simulink model "PippoSchema"  (R2022b)
settings: Solver=VariableStepAuto  StartTime=0.0  StopTime=2  RelTol=1e-3
settings Model: Creator=Stefano  LastModifiedBy=stefanopanzieri
settings SolverCC: AlgebraicLoopSolver=TrustRegion
settings OptimizationCC: ReuseModelBlockBuffer=on
settings DebuggingCC: UnconnectedInputMsg=warning  UnconnectedOutputMsg=warning  UnconnectedLineMsg=warning
settings ModelReferenceCC: EnableRefExpFcnMdlSchedulingChecks=on
settings SFSimCC: CustomCodeUndefinedFunction=UseInterfaceOnly
settings RTWCC: DLArmComputeVersion=19.05

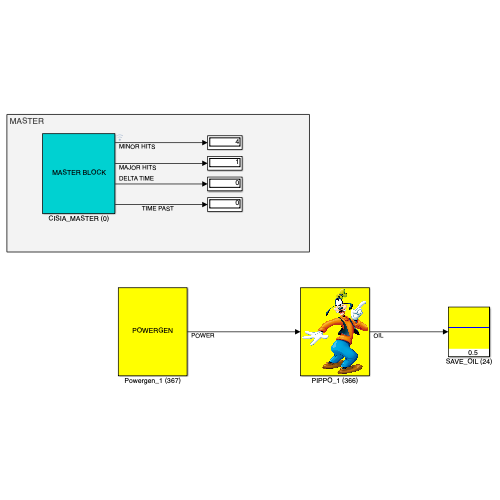
[thumbnail: Simulink's stored preview of the top-level diagram]
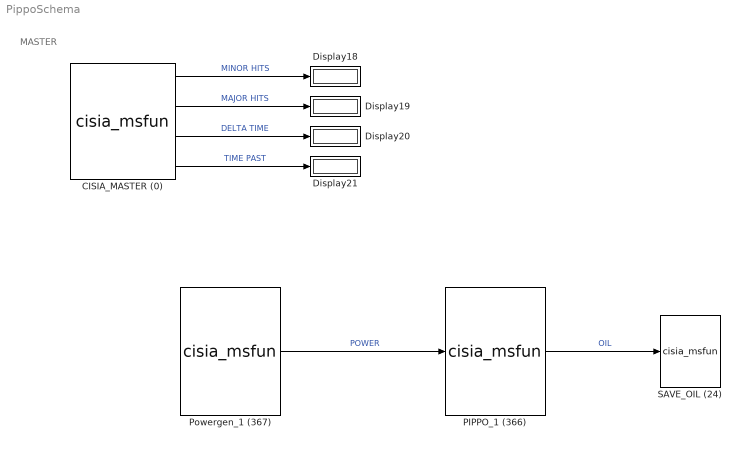
== system PippoSchema ==
  note: MASTER
  CISIA_MASTER (0) : M-S-Function  FunctionName=cisia_msfun  Parameters=Parameter1, Parameter2, Parameter3, resources, Parameter4, Parameter5, Parameter6, Parameter7, Parameter8, Parameter9,Parameter11  mask(S-function:msfcn_unit_delay){Parameter1='CISIA_MASTER', Parameter2=1, Parameter3='SistemiIoT', resources=off, Parameter4=on, Parameter5=off, Parameter6=off, Parameter7=off, Parameter8=0.001, Parameter9=off, Parameter11=on}
      mask prompts: Parameter1 "entity name"; Parameter2 "sampling time"; Parameter3 "project"; resources "Save status at each major hit"; Parameter4 "Show Operative Levels with colors"; Parameter5 "Load Entities from file"; Parameter6 "Load Start from Mask"; Parameter7 "Real Time"; Parameter8 "Real Time Hit (sec)"; Parameter9 "Skip saving"; Parameter11 "Show unconnected"
      mask help: This is a level-2 MATLAB file S-function which demonstrates CISIA entity
      mask Display: disp('MASTER BLOCK')
  Display{18..21} (4 alike) : Display
  PIPPO_1 (366) : M-S-Function  FunctionName=cisia_msfun  Parameters=Parameter1, Parameter2, Parameter3, resources, Parameter10, codeupdate, step_received, step_computed, dynamic_computed, step_sended, id_entity, id_project, id_type, name_type, color  mask(S-function:msfcn_unit_delay){Parameter1='PIPPO_1', Parameter2=1, Parameter3='', resources=|, Parameter10=off, codeupdate=off, step_received=Operative_Level=min([POWER  1-Mechanical_Fault]);, step_computed=, dynamic_computed=, step_sended=OIL=Operative_Level;, id_entity=366, id_project=6, id_type=100, name_type=PIPPO, color=#FFFFFF}
      mask resources=|
      | *** INPUT RESOURCES ***
      | NUM_INPUTS 1
      | POWER (1)
      |
      | *** STATE VARIABLES ***
      | NUM_VARIABLES 2
      | Operative_Level(NUMERIC)(1)(1)
      | Mechanical_Fault(NUMERIC)(1)(0)
      |
      | *** OUTPUT RESOURCES ***
      | NUM_OUTPUTS 1
      | OIL (1)
      mask prompts: Parameter1 "entity name"; Parameter2 "sampling time"; Parameter3 "project"; resources "input resources and state variables"; Parameter10 "Bring state variables to output"; codeupdate "update code from mask"
      mask help: This is a level-2 MATLAB file S-function which demonstrates CISIA entity
      mask DialogControl Container1 Prompt: All parameters
      mask Display: image('Icons/PIPPO.png')
  Powergen_1 (367) : M-S-Function  FunctionName=cisia_msfun  Parameters=Parameter1, Parameter2, Parameter3, resources, Parameter10, codeupdate, step_received, step_computed, dynamic_computed, step_sended, id_entity, id_project, id_type, name_type, color  mask(S-function:msfcn_unit_delay){Parameter1='Powergen_1', Parameter2=1, Parameter3='', resources=|, Parameter10=off, codeupdate=off, step_received=Operative_Level=1-Physical_Fault;, step_computed=, dynamic_computed=, step_sended=POWER=Operative_Level;, id_entity=367, id_project=6, id_type=101, name_type=POWERGEN, color=#FFFFFF}
      mask resources=|
      | *** INPUT RESOURCES ***
      | NUM_INPUTS 0
      |
      | *** STATE VARIABLES ***
      | NUM_VARIABLES 2
      | Operative_Level(NUMERIC)(1)(1)
      | Physical_Fault(NUMERIC)(1)(0.5)
      |
      | *** OUTPUT RESOURCES ***
      | NUM_OUTPUTS 1
      | POWER (1)
      mask prompts: Parameter1 "entity name"; Parameter2 "sampling time"; Parameter3 "project"; resources "input resources and state variables"; Parameter10 "Bring state variables to output"; codeupdate "update code from mask"
      mask help: This is a level-2 MATLAB file S-function which demonstrates CISIA entity
      mask DialogControl Container1 Prompt: All parameters
      mask Display: disp('POWERGEN')
  SAVE_OIL (24) : M-S-Function  FunctionName=cisia_msfun  Parameters=Parameter1, Parameter2, Parameter3, Parameter4,Parameter5,Parameter6,Parameter7  mask(S-function:msfcn_unit_delay){Parameter1='SAVE_OIL', Parameter2=1, Parameter3='SistemiIoT', Parameter4=on, Parameter5=[0.5], Parameter6=[1], Parameter7=off}
      mask prompts: Parameter1 "entity name"; Parameter2 "sampling time"; Parameter3 "project"; Parameter4 "display bars"; Parameter5 "values"; Parameter6 "logic"; Parameter7 "display B/W"
      mask help: This is a level-2 MATLAB file S-function which demonstrates CISIA entity
      mask DialogControl Container3 Prompt: Display
      mask Display:
      | display=get_param(gcb, 'Parameter4');
      | greymap=get_param(gcb, 'Parameter7');
      | 
      | if strcmp(display,'on')
      | 
      |     val=str2num(get_param(gcb, 'Parameter5'));
      |     logic=str2num(get_param(gcb, 'Parameter6'));
      |     n=length(val);
      | 
      |     val2=val;
      |     l=length(logic);
      |     if l>0
      |         for i=1:l
      |             if logic(i)==-1
      |                 val2(i)=1-val2(i);
      |             end
      |         end
      |     end
      | 
      | 
      | 
      | 
      |     if strcmp(greymap,'on')
      |         val_r=round(val2*50)+1;
      |         colormap=gray(60);
      |         color2=[0 0 0];
      |     else
      |         val_r=round(val2*20)+1;
      |         colormap=hsv(60);
      |         color2=[0 0 1];
      |     end
      | 
      |     patch([0 0 n n], [0 -0.2 -0.2 0], [1 1 1]);
      | 
      |     for i=1:n
      |         color=colormap(val_r(i),:);
      |         patch([i-1 i-1 i i],[0 1 1 0],color)
      |         patch([i-1 i],[val(i) val(i)],color2)
      | 
      |     end
      | 
      |     for i=1:n
      |         patch([i i], [-0.2 1], [0 0 0]);
      |         text(i-0.5, -0.1, num2str(val(i)));
      |     end
      | 
      | 
      | else
      | 
      |     disp('SAVE');
      | 
      | end
  wires:
  CISIA_MASTER (0)/1 -> Display18/1  "MINOR HITS"
  CISIA_MASTER (0)/2 -> Display19/1  "MAJOR HITS"
  CISIA_MASTER (0)/4 -> Display21/1  "TIME PAST"
  CISIA_MASTER (0)/3 -> Display20/1  "DELTA TIME"
  PIPPO_1 (366)/1 -> SAVE_OIL (24)/1  "OIL"
  Powergen_1 (367)/1 -> PIPPO_1 (366)/1  "POWER"
